simulink model "Scheduler"  (R2021b)
settings: Solver=VariableStepAuto  StartTime=0.0  StopTime=10.0  RelTol=1e-3
settings Model: Creator=fady  LastModifiedBy=fady

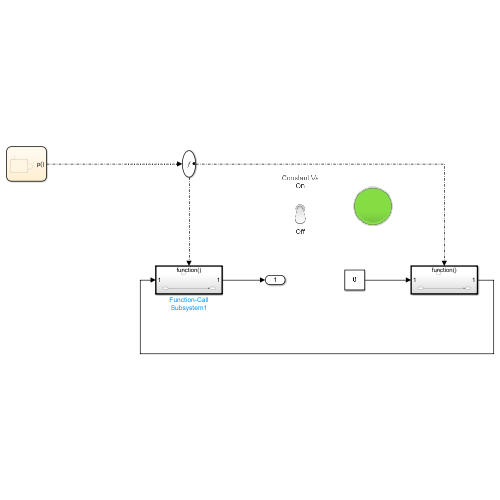
[thumbnail: Simulink's stored preview of the top-level diagram]
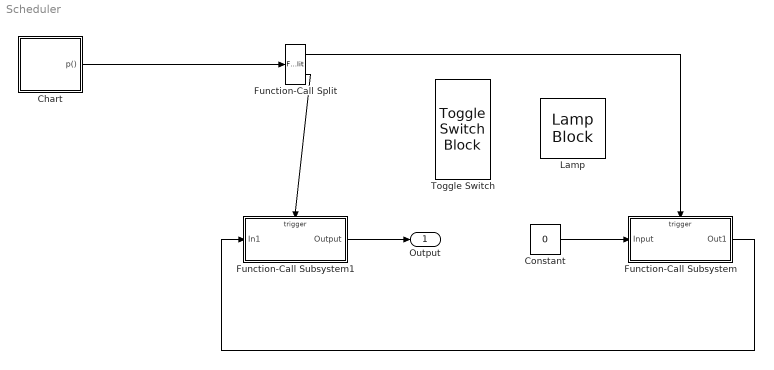
== system Scheduler ==
  Chart : Stateflow chart  TreatAsAtomicUnit=on
  Constant : Constant  Value=0
  Function-Call Split : FunctionCallSplit  NumOutputPorts=2  OutputPortLayout=default
  Function-Call Subsystem : Subsystem  TreatAsAtomicUnit=on
  Function-Call Subsystem1 : Subsystem  TreatAsAtomicUnit=on
  Lamp : LampBlock  LabelPosition=Hide
  Toggle Switch : ToggleSwitchBlock
      settings: Values={{'Off', 'On'}, [0 1]}
  Output : Outport
  wires:
  Chart/1(p()) -> Function-Call Split/1
  Function-Call Split/1 -> Function-Call Subsystem/Trigger
  Function-Call Split/2 -> Function-Call Subsystem1/Trigger
  Function-Call Subsystem/1(Out1) -> Function-Call Subsystem1/1(In1)
  Function-Call Subsystem1/1(Output) -> Output/1
  Constant/1 -> Function-Call Subsystem/1(Input)

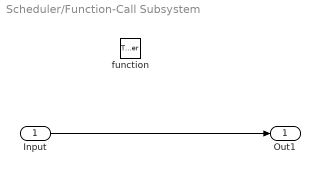
== system Scheduler/Function-Call Subsystem ==
  Input : Inport
  function : TriggerPort  TriggerType=function-call  VariantControl=(inherit)
  Out1 : Outport
  wires:
  Input/1 -> Out1/1

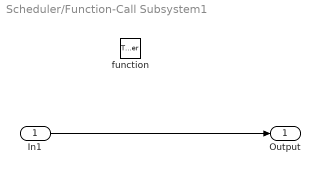
== system Scheduler/Function-Call Subsystem1 ==
  In1 : Inport
  function : TriggerPort  TriggerType=function-call  VariantControl=(inherit)
  Output : Outport
  wires:
  In1/1 -> Output/1

== stateflow chart Scheduler/Chart ==
  state Counter
    en:
    du:
    ex:
  (default) -> Counter
  Counter -> Counter : [after(5,tick)]{p;}
  events: p output FUNCTION_CALL_EVENT
